simulink model "Sys4"  (Simulink 6.6)
settings: Solver=ode45  StartTime=0.0  StopTime=time_span  RelTol=1e-3
undefined symbols (not defined in the file): K, noise_on, samp_time, Td, Ti
libraries: simulink_extras x2, simulink x1
settings Model: Creator=Jim  LastModifiedBy=Danai
settings DataIOCC: LimitDataPoints=off  SaveTime=off  TimeSaveName=t

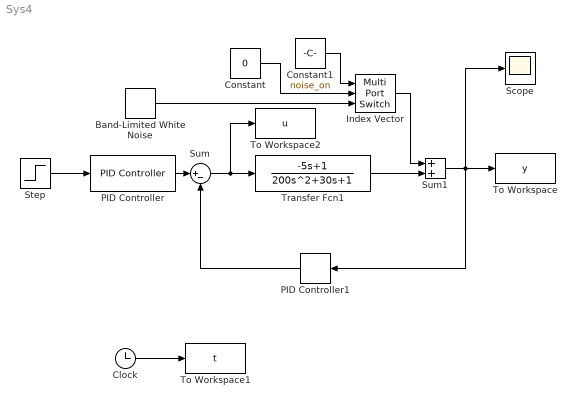
== system Sys4 ==
  Band-Limited White Noise : simulink/Sources/Band-Limited White Noise  SystemSampleTime=-1  Cov=[0.0001]  Ts=0.1  seed=[23341]
  Clock : Clock
      settings: Decimation=10
  Constant : Constant  Value=0
  Constant1 : Constant  Value=noise_on
  Index Vector : MultiPortSwitch  Inputs=2  zeroidx=on
  PID Controller : simulink_extras/Additional Linear/PID Controller  SystemSampleTime=-1  P=K  I=K/Ti  D=0
  PID Controller1 : simulink_extras/Additional Linear/PID Controller  Orientation=left  SystemSampleTime=-1  P=K  I=K/Ti  D=K*Td
  Scope : Scope
  Step : Step  Time=0  SampleTime=0
  Sum : Sum  Inputs=|+-
  Sum1 : Sum  Inputs=|++
  To Workspace : ToWorkspace  VariableName=y  SampleTime=samp_time  SaveFormat=Array
  To Workspace1 : ToWorkspace  VariableName=t  SampleTime=samp_time  SaveFormat=Array
  To Workspace2 : ToWorkspace  VariableName=u  SampleTime=samp_time  SaveFormat=Array
  Transfer Fcn1 : TransferFcn  Numerator=[-5 1]  Denominator=[200 30 1]
  wires:
  PID Controller1/1 -> Sum/2
  Sum/1 -> Transfer Fcn1/1, To Workspace2/1
  Sum1/1 -> To Workspace/1, Scope/1, PID Controller1/1
  Step/1 -> PID Controller/1
  PID Controller/1 -> Sum/1
  Transfer Fcn1/1 -> Sum1/2
  Index Vector/1 -> Sum1/1
  Constant1/1 -> Index Vector/1
  Constant/1 -> Index Vector/2
  Band-Limited White Noise/1 -> Index Vector/3
  Clock/1 -> To Workspace1/1
